simulink model "VAS_LEVEL1_TASK0_SETUP"  (Simulink 3.00)
undefined symbols (not defined in the file): data, dht, DHT_Z1, DHT_Z2, DHT_Z3, DHT_Z4, DHT_Z5, DHT_Z6, DHT_Z7, DHT_Z8, ephem, ephem_updater_bct, ephem_updater_ect, ephem_updater_moonrise, ephem_updater_moonset, ephem_updater_moontransit, ephem_updater_sunrise, ephem_updater_sunset, ephem_updater_suntransit, python, rex
libraries: mathlib x85, paramlib x18, logiclib x18, speclib x16, genlib x4, matrixlib x2, timelib x1

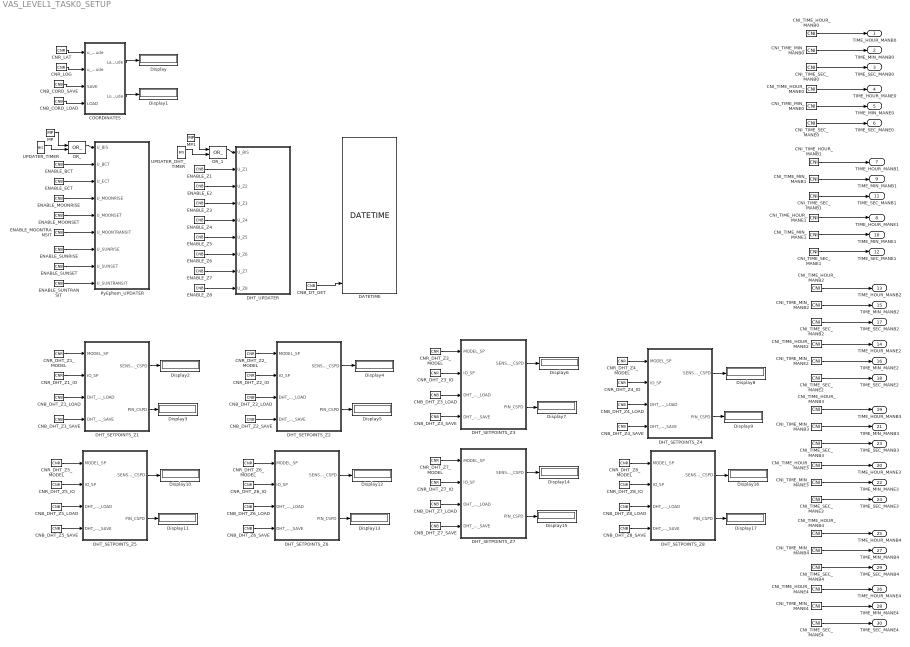
== system VAS_LEVEL1_TASK0_SETUP ==
  CNB_CORD_LOAD : mathlib/CNB  YCN=off
  CNB_CORD_SAVE : mathlib/CNB  YCN=off
  CNB_DHT_Z1_LOAD : mathlib/CNB  YCN=off
  CNB_DHT_Z1_SAVE : mathlib/CNB  YCN=off
  CNB_DHT_Z2_LOAD : mathlib/CNB  YCN=off
  CNB_DHT_Z2_SAVE : mathlib/CNB  YCN=off
  CNB_DHT_Z3_LOAD : mathlib/CNB  YCN=off
  CNB_DHT_Z3_SAVE : mathlib/CNB  YCN=off
  CNB_DHT_Z4_LOAD : mathlib/CNB  YCN=off
  CNB_DHT_Z4_SAVE : mathlib/CNB  YCN=off
  CNB_DHT_Z5_LOAD : mathlib/CNB  YCN=off
  CNB_DHT_Z5_SAVE : mathlib/CNB  YCN=off
  CNB_DHT_Z6_LOAD : mathlib/CNB  YCN=off
  CNB_DHT_Z6_SAVE : mathlib/CNB  YCN=off
  CNB_DHT_Z7_LOAD : mathlib/CNB  YCN=off
  CNB_DHT_Z7_SAVE : mathlib/CNB  YCN=off
  CNB_DHT_Z8_LOAD : mathlib/CNB  YCN=off
  CNB_DHT_Z8_SAVE : mathlib/CNB  YCN=off
  CNB_DT_GET : mathlib/CNB  YCN=off
  CNI_TIME_HOUR_MANB0 : mathlib/CNI  icn=20
  CNI_TIME_HOUR_MANB1 : mathlib/CNI  icn=14
  CNI_TIME_HOUR_MANB2 : mathlib/CNI  icn=16
  CNI_TIME_HOUR_MANB3 : mathlib/CNI  icn=18
  CNI_TIME_HOUR_MANB4 : mathlib/CNI  icn=0
  CNI_TIME_HOUR_MANE0 : mathlib/CNI  icn=22
  CNI_TIME_HOUR_MANE1 : mathlib/CNI  icn=16
  CNI_TIME_HOUR_MANE2 : mathlib/CNI  icn=18
  CNI_TIME_HOUR_MANE3 : mathlib/CNI  icn=20
  CNI_TIME_HOUR_MANE4 : mathlib/CNI  icn=0
  CNI_TIME_MIN_MANB{0..4} (5 alike) : mathlib/CNI  icn=0
  CNI_TIME_MIN_MANE{0..3} (4 alike) : mathlib/CNI  icn=0
  CNI_TIME_MIN_MANE4 : mathlib/CNI  icn=50
  CNI_TIME_SEC_MANB{0..4} (5 alike) : mathlib/CNI  icn=0
  CNI_TIME_SEC_MANE{0..4} (5 alike) : mathlib/CNI  icn=0
  CNR_DHT_Z1_IO : mathlib/CNR  ycn=5
  CNR_DHT_Z1_MODEL : mathlib/CNR  ycn=2
  CNR_DHT_Z2_IO : mathlib/CNR  ycn=6
  CNR_DHT_Z2_MODEL : mathlib/CNR  ycn=2
  CNR_DHT_Z3_IO : mathlib/CNR  ycn=16
  CNR_DHT_Z3_MODEL : mathlib/CNR  ycn=2
  CNR_DHT_Z4_IO : mathlib/CNR  ycn=17
  CNR_DHT_Z4_MODEL : mathlib/CNR  ycn=2
  CNR_DHT_Z5_IO : mathlib/CNR  ycn=0
  CNR_DHT_Z5_MODEL : mathlib/CNR  ycn=2
  CNR_DHT_Z6_IO : mathlib/CNR  ycn=0
  CNR_DHT_Z6_MODEL : mathlib/CNR  ycn=2
  CNR_DHT_Z7_IO : mathlib/CNR  ycn=0
  CNR_DHT_Z7_MODEL : mathlib/CNR  ycn=2
  CNR_DHT_Z8_IO : mathlib/CNR  ycn=0
  CNR_DHT_Z8_MODEL : mathlib/CNR  ycn=2
  CNR_LAT : mathlib/CNR  ycn=31.1729
  CNR_LOG : mathlib/CNR  ycn=-81.4772
  COORDINATES : Subsystem
      mask Type: REX sequence
  DATETIME : timelib/DATETIME  isetmode=6: The usec input - set HW clock only  igetmode=7: HW clock  settol=1  setper=0  getper=0.001  FDOW=off  tz=1: Local time
  DHT_SETPOINTS_Z1 : Subsystem
      mask Type: REX sequence
  DHT_SETPOINTS_Z2 : Subsystem
      mask Type: REX sequence
  DHT_SETPOINTS_Z3 : Subsystem
      mask Type: REX sequence
  DHT_SETPOINTS_Z4 : Subsystem
      mask Type: REX sequence
  DHT_SETPOINTS_Z5 : Subsystem
      mask Type: REX sequence
  DHT_SETPOINTS_Z6 : Subsystem
      mask Type: REX sequence
  DHT_SETPOINTS_Z7 : Subsystem
      mask Type: REX sequence
  DHT_SETPOINTS_Z8 : Subsystem
      mask Type: REX sequence
  DHT_UPDATER : Subsystem
      mask Type: REX sequence
  Display{,1..17} (18 alike) : Display
      settings: Format=Best fit
  ENABLE_BCT : mathlib/CNB  YCN=on
  ENABLE_E2 : mathlib/CNB  YCN=off
  ENABLE_ECT : mathlib/CNB  YCN=on
  ENABLE_MOONRISE : mathlib/CNB  YCN=on
  ENABLE_MOONSET : mathlib/CNB  YCN=on
  ENABLE_MOONTRANSIT : mathlib/CNB  YCN=on
  ENABLE_SUNRISE : mathlib/CNB  YCN=on
  ENABLE_SUNSET : mathlib/CNB  YCN=on
  ENABLE_SUNTRANSIT : mathlib/CNB  YCN=on
  ENABLE_Z{1,3..8} (7 alike) : mathlib/CNB  YCN=off
  MP : genlib/MP  BSTATE=on  pwidth=2  RPTF=off
  MP1 : genlib/MP  BSTATE=on  pwidth=2  RPTF=off
  OR_ : logiclib/OR_
  OR_1 : logiclib/OR_
  PyEphem_UPDATER : Subsystem
      mask Type: REX sequence
  UPDATER_DHT_TIMER : genlib/BIS  Y0=off  t1=0  t2=1  t3=15  t4=4  t5=5  t6=6  t7=7  t8=8  RPT=on  bEdit=off
  UPDATER_TIMER : genlib/BIS  Y0=off  t1=0  t2=1  t3=3600  t4=4  t5=5  t6=6  t7=7  t8=8  RPT=on  bEdit=off
  TIME_HOUR_MANB0 : Outport  Port=1
  TIME_MIN_MANB0 : Outport  Port=2
  TIME_SEC_MANB0 : Outport  Port=3
  TIME_HOUR_MANE0 : Outport  Port=4
  TIME_MIN_MANE0 : Outport  Port=5
  TIME_SEC_MANE0 : Outport  Port=6
  TIME_HOUR_MANB1 : Outport  Port=7
  TIME_HOUR_MANE1 : Outport  Port=8
  TIME_MIN_MANB1 : Outport  Port=9
  TIME_MIN_MANE1 : Outport  Port=10
  TIME_SEC_MANB1 : Outport  Port=11
  TIME_SEC_MANE1 : Outport  Port=12
  TIME_HOUR_MANB2 : Outport  Port=13
  TIME_HOUR_MANE2 : Outport  Port=14
  TIME_MIN_MANB2 : Outport  Port=15
  TIME_MIN_MANE2 : Outport  Port=16
  TIME_SEC_MANB2 : Outport  Port=17
  TIME_SEC_MANE2 : Outport  Port=18
  TIME_HOUR_MANB3 : Outport  Port=19
  TIME_HOUR_MANE3 : Outport  Port=20
  TIME_MIN_MANB3 : Outport  Port=21
  TIME_MIN_MANE3 : Outport  Port=22
  TIME_SEC_MANB3 : Outport  Port=23
  TIME_SEC_MANE3 : Outport  Port=24
  TIME_HOUR_MANB4 : Outport  Port=25
  TIME_HOUR_MANE4 : Outport  Port=26
  TIME_MIN_MANB4 : Outport  Port=27
  TIME_MIN_MANE4 : Outport  Port=28
  TIME_SEC_MANB4 : Outport  Port=29
  TIME_SEC_MANE4 : Outport  Port=30
  wires:
  CNB_CORD_LOAD/1 -> COORDINATES/4(LOAD)
  CNB_CORD_SAVE/1 -> COORDINATES/3(SAVE)
  CNB_DHT_Z1_LOAD/1 -> DHT_SETPOINTS_Z1/3(DHT_MIO_LOAD)
  CNB_DHT_Z1_SAVE/1 -> DHT_SETPOINTS_Z1/4(DHT_MIO_SAVE)
  CNB_DHT_Z2_LOAD/1 -> DHT_SETPOINTS_Z2/3(DHT_MIO_LOAD)
  CNB_DHT_Z2_SAVE/1 -> DHT_SETPOINTS_Z2/4(DHT_MIO_SAVE)
  CNB_DHT_Z3_LOAD/1 -> DHT_SETPOINTS_Z3/3(DHT_MIO_LOAD)
  CNB_DHT_Z3_SAVE/1 -> DHT_SETPOINTS_Z3/4(DHT_MIO_SAVE)
  CNB_DHT_Z4_LOAD/1 -> DHT_SETPOINTS_Z4/3(DHT_MIO_LOAD)
  CNB_DHT_Z4_SAVE/1 -> DHT_SETPOINTS_Z4/4(DHT_MIO_SAVE)
  CNB_DHT_Z5_LOAD/1 -> DHT_SETPOINTS_Z5/3(DHT_MIO_LOAD)
  CNB_DHT_Z5_SAVE/1 -> DHT_SETPOINTS_Z5/4(DHT_MIO_SAVE)
  CNB_DHT_Z6_LOAD/1 -> DHT_SETPOINTS_Z6/3(DHT_MIO_LOAD)
  CNB_DHT_Z6_SAVE/1 -> DHT_SETPOINTS_Z6/4(DHT_MIO_SAVE)
  CNB_DHT_Z7_LOAD/1 -> DHT_SETPOINTS_Z7/3(DHT_MIO_LOAD)
  CNB_DHT_Z7_SAVE/1 -> DHT_SETPOINTS_Z7/4(DHT_MIO_SAVE)
  CNB_DHT_Z8_LOAD/1 -> DHT_SETPOINTS_Z8/3(DHT_MIO_LOAD)
  CNB_DHT_Z8_SAVE/1 -> DHT_SETPOINTS_Z8/4(DHT_MIO_SAVE)
  CNB_DT_GET/1 -> DATETIME/9
  CNI_TIME_HOUR_MANB0/1 -> TIME_HOUR_MANB0/1
  CNI_TIME_HOUR_MANB1/1 -> TIME_HOUR_MANB1/1
  CNI_TIME_HOUR_MANB2/1 -> TIME_HOUR_MANB2/1
  CNI_TIME_HOUR_MANB3/1 -> TIME_HOUR_MANB3/1
  CNI_TIME_HOUR_MANB4/1 -> TIME_HOUR_MANB4/1
  CNI_TIME_HOUR_MANE0/1 -> TIME_HOUR_MANE0/1
  CNI_TIME_HOUR_MANE1/1 -> TIME_HOUR_MANE1/1
  CNI_TIME_HOUR_MANE2/1 -> TIME_HOUR_MANE2/1
  CNI_TIME_HOUR_MANE3/1 -> TIME_HOUR_MANE3/1
  CNI_TIME_HOUR_MANE4/1 -> TIME_HOUR_MANE4/1
  CNI_TIME_MIN_MANB0/1 -> TIME_MIN_MANB0/1
  CNI_TIME_MIN_MANB1/1 -> TIME_MIN_MANB1/1
  CNI_TIME_MIN_MANB2/1 -> TIME_MIN_MANB2/1
  CNI_TIME_MIN_MANB3/1 -> TIME_MIN_MANB3/1
  CNI_TIME_MIN_MANB4/1 -> TIME_MIN_MANB4/1
  CNI_TIME_MIN_MANE0/1 -> TIME_MIN_MANE0/1
  CNI_TIME_MIN_MANE1/1 -> TIME_MIN_MANE1/1
  CNI_TIME_MIN_MANE2/1 -> TIME_MIN_MANE2/1
  CNI_TIME_MIN_MANE3/1 -> TIME_MIN_MANE3/1
  CNI_TIME_MIN_MANE4/1 -> TIME_MIN_MANE4/1
  CNI_TIME_SEC_MANB0/1 -> TIME_SEC_MANB0/1
  CNI_TIME_SEC_MANB1/1 -> TIME_SEC_MANB1/1
  CNI_TIME_SEC_MANB2/1 -> TIME_SEC_MANB2/1
  CNI_TIME_SEC_MANB3/1 -> TIME_SEC_MANB3/1
  CNI_TIME_SEC_MANB4/1 -> TIME_SEC_MANB4/1
  CNI_TIME_SEC_MANE0/1 -> TIME_SEC_MANE0/1
  CNI_TIME_SEC_MANE1/1 -> TIME_SEC_MANE1/1
  CNI_TIME_SEC_MANE2/1 -> TIME_SEC_MANE2/1
  CNI_TIME_SEC_MANE3/1 -> TIME_SEC_MANE3/1
  CNI_TIME_SEC_MANE4/1 -> TIME_SEC_MANE4/1
  CNR_DHT_Z1_IO/1 -> DHT_SETPOINTS_Z1/2(IO_SP)
  CNR_DHT_Z1_MODEL/1 -> DHT_SETPOINTS_Z1/1(MODEL_SP)
  CNR_DHT_Z2_IO/1 -> DHT_SETPOINTS_Z2/2(IO_SP)
  CNR_DHT_Z2_MODEL/1 -> DHT_SETPOINTS_Z2/1(MODEL_SP)
  CNR_DHT_Z3_IO/1 -> DHT_SETPOINTS_Z3/2(IO_SP)
  CNR_DHT_Z3_MODEL/1 -> DHT_SETPOINTS_Z3/1(MODEL_SP)
  CNR_DHT_Z4_IO/1 -> DHT_SETPOINTS_Z4/2(IO_SP)
  CNR_DHT_Z4_MODEL/1 -> DHT_SETPOINTS_Z4/1(MODEL_SP)
  CNR_DHT_Z5_IO/1 -> DHT_SETPOINTS_Z5/2(IO_SP)
  CNR_DHT_Z5_MODEL/1 -> DHT_SETPOINTS_Z5/1(MODEL_SP)
  CNR_DHT_Z6_IO/1 -> DHT_SETPOINTS_Z6/2(IO_SP)
  CNR_DHT_Z6_MODEL/1 -> DHT_SETPOINTS_Z6/1(MODEL_SP)
  CNR_DHT_Z7_IO/1 -> DHT_SETPOINTS_Z7/2(IO_SP)
  CNR_DHT_Z7_MODEL/1 -> DHT_SETPOINTS_Z7/1(MODEL_SP)
  CNR_DHT_Z8_IO/1 -> DHT_SETPOINTS_Z8/2(IO_SP)
  CNR_DHT_Z8_MODEL/1 -> DHT_SETPOINTS_Z8/1(MODEL_SP)
  CNR_LAT/1 -> COORDINATES/1(u_Latitude)
  CNR_LOG/1 -> COORDINATES/2(u_Longitude)
  COORDINATES/1(Latitude) -> Display/1
  COORDINATES/2(Longitude) -> Display1/1
  DHT_SETPOINTS_Z1/1(SENSOR_CSPD) -> Display2/1
  DHT_SETPOINTS_Z1/2(PIN_CSPD) -> Display3/1
  DHT_SETPOINTS_Z2/1(SENSOR_CSPD) -> Display4/1
  DHT_SETPOINTS_Z2/2(PIN_CSPD) -> Display5/1
  DHT_SETPOINTS_Z3/1(SENSOR_CSPD) -> Display6/1
  DHT_SETPOINTS_Z3/2(PIN_CSPD) -> Display7/1
  DHT_SETPOINTS_Z4/1(SENSOR_CSPD) -> Display8/1
  DHT_SETPOINTS_Z4/2(PIN_CSPD) -> Display9/1
  DHT_SETPOINTS_Z5/1(SENSOR_CSPD) -> Display10/1
  DHT_SETPOINTS_Z5/2(PIN_CSPD) -> Display11/1
  DHT_SETPOINTS_Z6/1(SENSOR_CSPD) -> Display12/1
  DHT_SETPOINTS_Z6/2(PIN_CSPD) -> Display13/1
  DHT_SETPOINTS_Z7/1(SENSOR_CSPD) -> Display14/1
  DHT_SETPOINTS_Z7/2(PIN_CSPD) -> Display15/1
  DHT_SETPOINTS_Z8/1(SENSOR_CSPD) -> Display16/1
  DHT_SETPOINTS_Z8/2(PIN_CSPD) -> Display17/1
  ENABLE_BCT/1 -> PyEphem_UPDATER/2(U_BCT)
  ENABLE_E2/1 -> DHT_UPDATER/3(U_Z2)
  ENABLE_ECT/1 -> PyEphem_UPDATER/3(U_ECT)
  ENABLE_MOONRISE/1 -> PyEphem_UPDATER/4(U_MOONRISE)
  ENABLE_MOONSET/1 -> PyEphem_UPDATER/5(U_MOONSET)
  ENABLE_MOONTRANSIT/1 -> PyEphem_UPDATER/6(U_MOONTRANSIT)
  ENABLE_SUNRISE/1 -> PyEphem_UPDATER/7(U_SUNRISE)
  ENABLE_SUNSET/1 -> PyEphem_UPDATER/8(U_SUNSET)
  ENABLE_SUNTRANSIT/1 -> PyEphem_UPDATER/9(U_SUNTRANSIT)
  ENABLE_Z1/1 -> DHT_UPDATER/2(U_Z1)
  ENABLE_Z3/1 -> DHT_UPDATER/4(U_Z3)
  ENABLE_Z4/1 -> DHT_UPDATER/5(U_Z4)
  ENABLE_Z5/1 -> DHT_UPDATER/6(U_Z5)
  ENABLE_Z6/1 -> DHT_UPDATER/7(U_Z6)
  ENABLE_Z7/1 -> DHT_UPDATER/8(U_Z7)
  ENABLE_Z8/1 -> DHT_UPDATER/9(U_Z8)
  MP/1 -> OR_/1
  MP1/1 -> OR_1/1
  OR_/1 -> PyEphem_UPDATER/1(U_BIS)
  OR_1/1 -> DHT_UPDATER/1(U_BIS)
  UPDATER_DHT_TIMER/1 -> OR_1/2
  UPDATER_TIMER/1 -> OR_/2

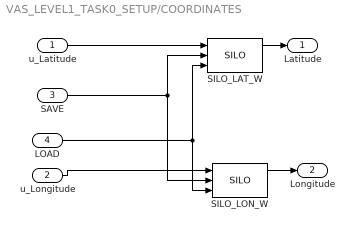
== system VAS_LEVEL1_TASK0_SETUP/COORDINATES ==
  u_Latitude : Inport  Port=1
  u_Longitude : Inport  Port=2
  SAVE : Inport  Port=3
  LOAD : Inport  Port=4
  SILO_LAT_W : paramlib/SILO  fname=/static/LAT.txt  CSF=off  CLF=off  yerr=0
  SILO_LON_W : paramlib/SILO  fname=/static/LON.txt  CSF=off  CLF=off  yerr=0
  Latitude : Outport  Port=1
  Longitude : Outport  Port=2
  wires:
  LOAD/1 -> SILO_LAT_W/3, SILO_LON_W/3
  SAVE/1 -> SILO_LAT_W/2, SILO_LON_W/2
  SILO_LAT_W/1 -> Latitude/1
  SILO_LON_W/1 -> Longitude/1
  u_Latitude/1 -> SILO_LAT_W/1
  u_Longitude/1 -> SILO_LON_W/1

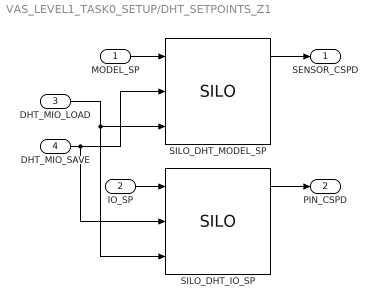
== system VAS_LEVEL1_TASK0_SETUP/DHT_SETPOINTS_Z1 ==
  MODEL_SP : Inport  Port=1
  IO_SP : Inport  Port=2
  DHT_MIO_LOAD : Inport  Port=3
  DHT_MIO_SAVE : Inport  Port=4
  SILO_DHT_IO_SP : paramlib/SILO  fname=/static/DHT_Z1_PIN.txt  CSF=off  CLF=off  yerr=0
  SILO_DHT_MODEL_SP : paramlib/SILO  fname=/static/DHT_Z1_SENSOR.txt  CSF=off  CLF=off  yerr=0
  SENSOR_CSPD : Outport  Port=1
  PIN_CSPD : Outport  Port=2
  wires:
  DHT_MIO_LOAD/1 -> SILO_DHT_IO_SP/3, SILO_DHT_MODEL_SP/3
  DHT_MIO_SAVE/1 -> SILO_DHT_IO_SP/2, SILO_DHT_MODEL_SP/2
  IO_SP/1 -> SILO_DHT_IO_SP/1
  MODEL_SP/1 -> SILO_DHT_MODEL_SP/1
  SILO_DHT_IO_SP/1 -> PIN_CSPD/1
  SILO_DHT_MODEL_SP/1 -> SENSOR_CSPD/1

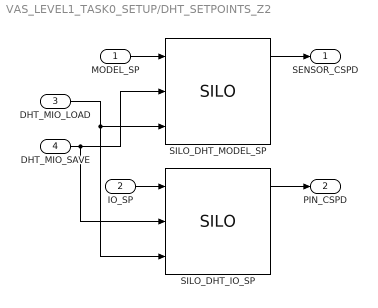
== system VAS_LEVEL1_TASK0_SETUP/DHT_SETPOINTS_Z2 ==
  MODEL_SP : Inport  Port=1
  IO_SP : Inport  Port=2
  DHT_MIO_LOAD : Inport  Port=3
  DHT_MIO_SAVE : Inport  Port=4
  SILO_DHT_IO_SP : paramlib/SILO  fname=/static/DHT_Z2_PIN.txt  CSF=off  CLF=off  yerr=0
  SILO_DHT_MODEL_SP : paramlib/SILO  fname=/static/DHT_Z2_SENSOR.txt  CSF=off  CLF=off  yerr=0
  SENSOR_CSPD : Outport  Port=1
  PIN_CSPD : Outport  Port=2
  wires:
  DHT_MIO_LOAD/1 -> SILO_DHT_IO_SP/3, SILO_DHT_MODEL_SP/3
  DHT_MIO_SAVE/1 -> SILO_DHT_IO_SP/2, SILO_DHT_MODEL_SP/2
  IO_SP/1 -> SILO_DHT_IO_SP/1
  MODEL_SP/1 -> SILO_DHT_MODEL_SP/1
  SILO_DHT_IO_SP/1 -> PIN_CSPD/1
  SILO_DHT_MODEL_SP/1 -> SENSOR_CSPD/1

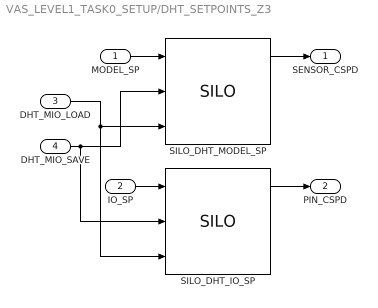
== system VAS_LEVEL1_TASK0_SETUP/DHT_SETPOINTS_Z3 ==
  MODEL_SP : Inport  Port=1
  IO_SP : Inport  Port=2
  DHT_MIO_LOAD : Inport  Port=3
  DHT_MIO_SAVE : Inport  Port=4
  SILO_DHT_IO_SP : paramlib/SILO  fname=/static/DHT_Z3_PIN.txt  CSF=off  CLF=off  yerr=0
  SILO_DHT_MODEL_SP : paramlib/SILO  fname=/static/DHT_Z3_SENSOR.txt  CSF=off  CLF=off  yerr=0
  SENSOR_CSPD : Outport  Port=1
  PIN_CSPD : Outport  Port=2
  wires:
  DHT_MIO_LOAD/1 -> SILO_DHT_IO_SP/3, SILO_DHT_MODEL_SP/3
  DHT_MIO_SAVE/1 -> SILO_DHT_IO_SP/2, SILO_DHT_MODEL_SP/2
  IO_SP/1 -> SILO_DHT_IO_SP/1
  MODEL_SP/1 -> SILO_DHT_MODEL_SP/1
  SILO_DHT_IO_SP/1 -> PIN_CSPD/1
  SILO_DHT_MODEL_SP/1 -> SENSOR_CSPD/1

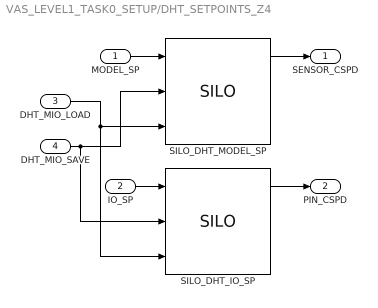
== system VAS_LEVEL1_TASK0_SETUP/DHT_SETPOINTS_Z4 ==
  MODEL_SP : Inport  Port=1
  IO_SP : Inport  Port=2
  DHT_MIO_LOAD : Inport  Port=3
  DHT_MIO_SAVE : Inport  Port=4
  SILO_DHT_IO_SP : paramlib/SILO  fname=/static/DHT_Z4_PIN.txt  CSF=off  CLF=off  yerr=0
  SILO_DHT_MODEL_SP : paramlib/SILO  fname=/static/DHT_Z4_SENSOR.txt  CSF=off  CLF=off  yerr=0
  SENSOR_CSPD : Outport  Port=1
  PIN_CSPD : Outport  Port=2
  wires:
  DHT_MIO_LOAD/1 -> SILO_DHT_IO_SP/3, SILO_DHT_MODEL_SP/3
  DHT_MIO_SAVE/1 -> SILO_DHT_IO_SP/2, SILO_DHT_MODEL_SP/2
  IO_SP/1 -> SILO_DHT_IO_SP/1
  MODEL_SP/1 -> SILO_DHT_MODEL_SP/1
  SILO_DHT_IO_SP/1 -> PIN_CSPD/1
  SILO_DHT_MODEL_SP/1 -> SENSOR_CSPD/1

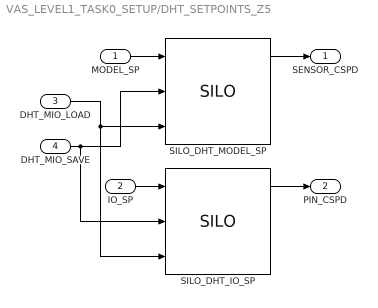
== system VAS_LEVEL1_TASK0_SETUP/DHT_SETPOINTS_Z5 ==
  MODEL_SP : Inport  Port=1
  IO_SP : Inport  Port=2
  DHT_MIO_LOAD : Inport  Port=3
  DHT_MIO_SAVE : Inport  Port=4
  SILO_DHT_IO_SP : paramlib/SILO  fname=/static/DHT_Z5_PIN.txt  CSF=off  CLF=off  yerr=0
  SILO_DHT_MODEL_SP : paramlib/SILO  fname=/static/DHT_Z5_SENSOR.txt  CSF=off  CLF=off  yerr=0
  SENSOR_CSPD : Outport  Port=1
  PIN_CSPD : Outport  Port=2
  wires:
  DHT_MIO_LOAD/1 -> SILO_DHT_IO_SP/3, SILO_DHT_MODEL_SP/3
  DHT_MIO_SAVE/1 -> SILO_DHT_IO_SP/2, SILO_DHT_MODEL_SP/2
  IO_SP/1 -> SILO_DHT_IO_SP/1
  MODEL_SP/1 -> SILO_DHT_MODEL_SP/1
  SILO_DHT_IO_SP/1 -> PIN_CSPD/1
  SILO_DHT_MODEL_SP/1 -> SENSOR_CSPD/1

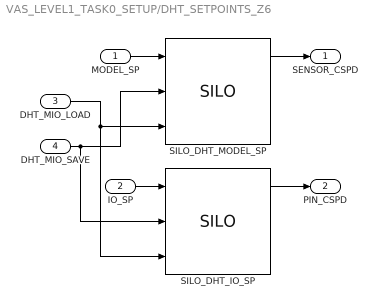
== system VAS_LEVEL1_TASK0_SETUP/DHT_SETPOINTS_Z6 ==
  MODEL_SP : Inport  Port=1
  IO_SP : Inport  Port=2
  DHT_MIO_LOAD : Inport  Port=3
  DHT_MIO_SAVE : Inport  Port=4
  SILO_DHT_IO_SP : paramlib/SILO  fname=/static/DHT_Z6_PIN.txt  CSF=off  CLF=off  yerr=0
  SILO_DHT_MODEL_SP : paramlib/SILO  fname=/static/DHT_Z6_SENSOR.txt  CSF=off  CLF=off  yerr=0
  SENSOR_CSPD : Outport  Port=1
  PIN_CSPD : Outport  Port=2
  wires:
  DHT_MIO_LOAD/1 -> SILO_DHT_IO_SP/3, SILO_DHT_MODEL_SP/3
  DHT_MIO_SAVE/1 -> SILO_DHT_IO_SP/2, SILO_DHT_MODEL_SP/2
  IO_SP/1 -> SILO_DHT_IO_SP/1
  MODEL_SP/1 -> SILO_DHT_MODEL_SP/1
  SILO_DHT_IO_SP/1 -> PIN_CSPD/1
  SILO_DHT_MODEL_SP/1 -> SENSOR_CSPD/1

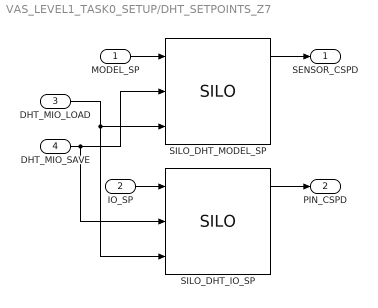
== system VAS_LEVEL1_TASK0_SETUP/DHT_SETPOINTS_Z7 ==
  MODEL_SP : Inport  Port=1
  IO_SP : Inport  Port=2
  DHT_MIO_LOAD : Inport  Port=3
  DHT_MIO_SAVE : Inport  Port=4
  SILO_DHT_IO_SP : paramlib/SILO  fname=/static/DHT_Z7_PIN.txt  CSF=off  CLF=off  yerr=0
  SILO_DHT_MODEL_SP : paramlib/SILO  fname=/static/DHT_Z7_SENSOR.txt  CSF=off  CLF=off  yerr=0
  SENSOR_CSPD : Outport  Port=1
  PIN_CSPD : Outport  Port=2
  wires:
  DHT_MIO_LOAD/1 -> SILO_DHT_IO_SP/3, SILO_DHT_MODEL_SP/3
  DHT_MIO_SAVE/1 -> SILO_DHT_IO_SP/2, SILO_DHT_MODEL_SP/2
  IO_SP/1 -> SILO_DHT_IO_SP/1
  MODEL_SP/1 -> SILO_DHT_MODEL_SP/1
  SILO_DHT_IO_SP/1 -> PIN_CSPD/1
  SILO_DHT_MODEL_SP/1 -> SENSOR_CSPD/1

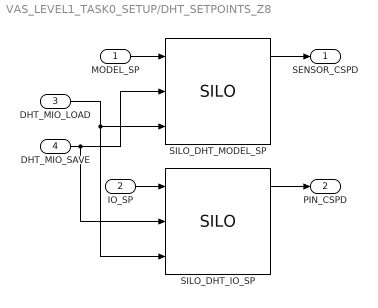
== system VAS_LEVEL1_TASK0_SETUP/DHT_SETPOINTS_Z8 ==
  MODEL_SP : Inport  Port=1
  IO_SP : Inport  Port=2
  DHT_MIO_LOAD : Inport  Port=3
  DHT_MIO_SAVE : Inport  Port=4
  SILO_DHT_IO_SP : paramlib/SILO  fname=/static/DHT_Z8_PIN.txt  CSF=off  CLF=off  yerr=0
  SILO_DHT_MODEL_SP : paramlib/SILO  fname=/static/DHT_Z8_SENSOR.txt  CSF=off  CLF=off  yerr=0
  SENSOR_CSPD : Outport  Port=1
  PIN_CSPD : Outport  Port=2
  wires:
  DHT_MIO_LOAD/1 -> SILO_DHT_IO_SP/3, SILO_DHT_MODEL_SP/3
  DHT_MIO_SAVE/1 -> SILO_DHT_IO_SP/2, SILO_DHT_MODEL_SP/2
  IO_SP/1 -> SILO_DHT_IO_SP/1
  MODEL_SP/1 -> SILO_DHT_MODEL_SP/1
  SILO_DHT_IO_SP/1 -> PIN_CSPD/1
  SILO_DHT_MODEL_SP/1 -> SENSOR_CSPD/1

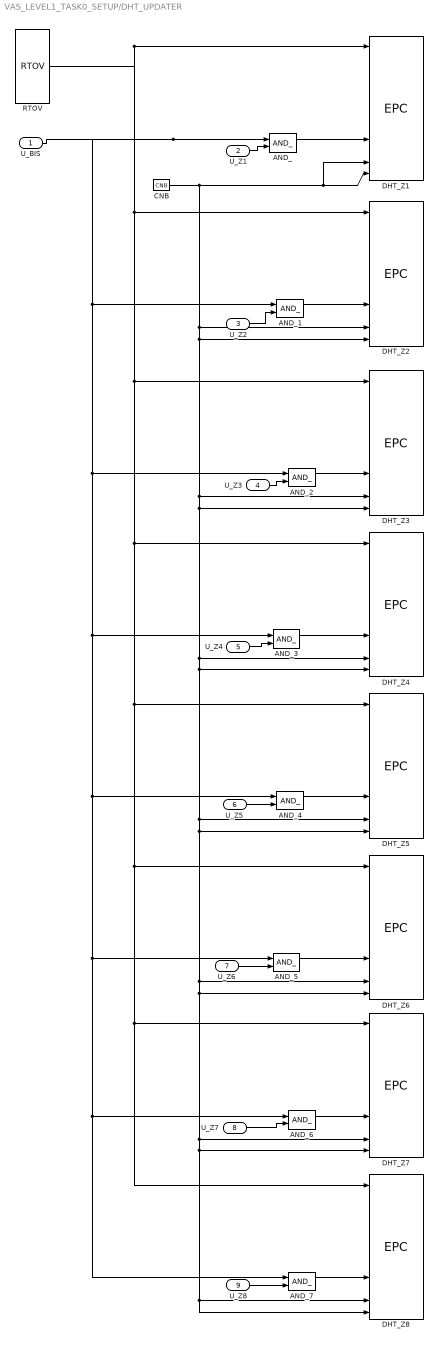
== system VAS_LEVEL1_TASK0_SETUP/DHT_UPDATER ==
  U_BIS : Inport  Port=1
  U_Z1 : Inport  Port=2
  U_Z2 : Inport  Port=3
  U_Z3 : Inport  Port=4
  U_Z4 : Inport  Port=5
  U_Z5 : Inport  Port=6
  U_Z6 : Inport  Port=7
  U_Z7 : Inport  Port=8
  U_Z8 : Inport  Port=9
  AND_{,1..7} (8 alike) : logiclib/AND_
  CNB : mathlib/CNB  YCN=off
  DHT_Z1 : speclib/EPC  cmd=python /rex/data/dht/DHT_Z1.py  sl=0  ifm=1  format=1: Space-delimited values  nmax=2
  DHT_Z2 : speclib/EPC  cmd=python /rex/data/dht/DHT_Z2.py  sl=0  ifm=1  format=1: Space-delimited values  nmax=2
  DHT_Z3 : speclib/EPC  cmd=python /rex/data/dht/DHT_Z3.py  sl=0  ifm=1  format=1: Space-delimited values  nmax=2
  DHT_Z4 : speclib/EPC  cmd=python /rex/data/dht/DHT_Z4.py  sl=0  ifm=1  format=1: Space-delimited values  nmax=2
  DHT_Z5 : speclib/EPC  cmd=python /rex/data/dht/DHT_Z5.py  sl=0  ifm=1  format=1: Space-delimited values  nmax=2
  DHT_Z6 : speclib/EPC  cmd=python /rex/data/dht/DHT_Z6.py  sl=0  ifm=1  format=1: Space-delimited values  nmax=2
  DHT_Z7 : speclib/EPC  cmd=python /rex/data/dht/DHT_Z7.py  sl=0  ifm=1  format=1: Space-delimited values  nmax=2
  DHT_Z8 : speclib/EPC  cmd=python /rex/data/dht/DHT_Z8.py  sl=0  ifm=1  format=1: Space-delimited values  nmax=2
  RTOV : matrixlib/RTOV  nmax=8  offset=0  n=8  etype=8: Double
  wires:
  AND_/1 -> DHT_Z1/9
  AND_1/1 -> DHT_Z2/9
  AND_2/1 -> DHT_Z3/9
  AND_3/1 -> DHT_Z4/9
  AND_4/1 -> DHT_Z5/9
  AND_5/1 -> DHT_Z6/9
  AND_6/1 -> DHT_Z7/9
  AND_7/1 -> DHT_Z8/9
  CNB/1 -> DHT_Z1/11, DHT_Z1/12, DHT_Z2/11, DHT_Z2/12, DHT_Z3/11, DHT_Z3/12, DHT_Z4/11, DHT_Z4/12, DHT_Z5/11, DHT_Z5/12, DHT_Z6/11, DHT_Z6/12, DHT_Z7/11, DHT_Z7/12, DHT_Z8/11, DHT_Z8/12
  RTOV/1 -> DHT_Z1/1, DHT_Z2/1, DHT_Z7/1, DHT_Z8/1, DHT_Z6/1, DHT_Z5/1, DHT_Z4/1, DHT_Z3/1
  U_BIS/1 -> AND_/1, AND_1/1, AND_5/1, AND_6/1, AND_7/1, AND_4/1, AND_3/1, AND_2/1
  U_Z1/1 -> AND_/2
  U_Z2/1 -> AND_1/2
  U_Z3/1 -> AND_2/2
  U_Z4/1 -> AND_3/2
  U_Z5/1 -> AND_4/2
  U_Z6/1 -> AND_5/2
  U_Z7/1 -> AND_6/2
  U_Z8/1 -> AND_7/2

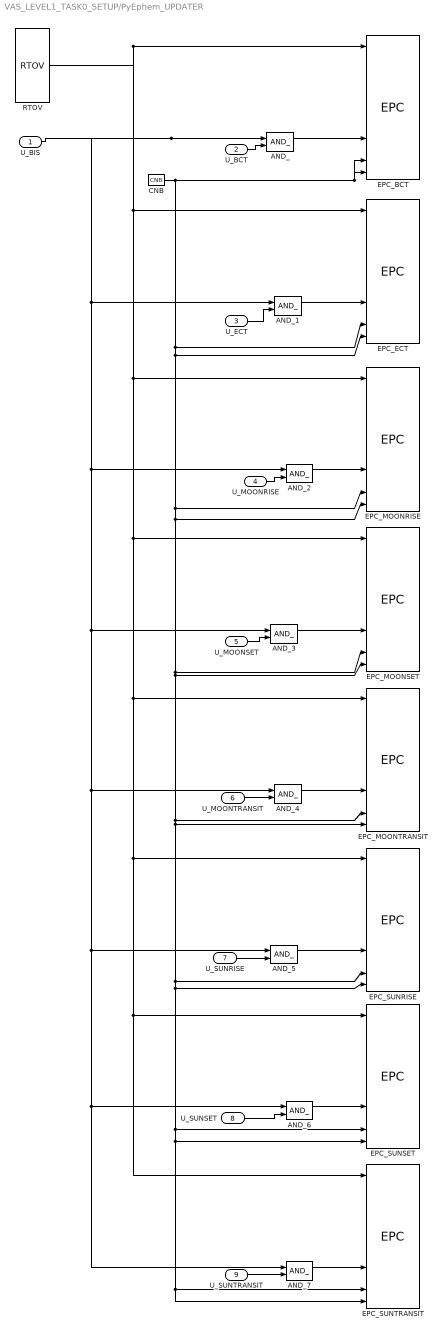
== system VAS_LEVEL1_TASK0_SETUP/PyEphem_UPDATER ==
  U_BIS : Inport  Port=1
  U_BCT : Inport  Port=2
  U_ECT : Inport  Port=3
  U_MOONRISE : Inport  Port=4
  U_MOONSET : Inport  Port=5
  U_MOONTRANSIT : Inport  Port=6
  U_SUNRISE : Inport  Port=7
  U_SUNSET : Inport  Port=8
  U_SUNTRANSIT : Inport  Port=9
  AND_{,1..7} (8 alike) : logiclib/AND_
  CNB : mathlib/CNB  YCN=off
  EPC_BCT : speclib/EPC  cmd=python /rex/data/ephem/ephem_updater_bct.py  sl=0  ifm=1  format=1: Space-delimited values  nmax=2
  EPC_ECT : speclib/EPC  cmd=python /rex/data/ephem/ephem_updater_ect.py  sl=0  ifm=1  format=1: Space-delimited values  nmax=2
  EPC_MOONRISE : speclib/EPC  cmd=python /rex/data/ephem/ephem_updater_moonrise.py  sl=0  ifm=1  format=1: Space-delimited values  nmax=2
  EPC_MOONSET : speclib/EPC  cmd=python /rex/data/ephem/ephem_updater_moonset.py  sl=0  ifm=1  format=1: Space-delimited values  nmax=2
  EPC_MOONTRANSIT : speclib/EPC  cmd=python /rex/data/ephem/ephem_updater_moontransit.py  sl=0  format=1: Space-delimited values  nmax=2
  EPC_SUNRISE : speclib/EPC  cmd=python /rex/data/ephem/ephem_updater_sunrise.py  sl=0  ifm=1  format=1: Space-delimited values  nmax=2
  EPC_SUNSET : speclib/EPC  cmd=python /rex/data/ephem/ephem_updater_sunset.py  sl=0  ifm=1  format=1: Space-delimited values  nmax=2
  EPC_SUNTRANSIT : speclib/EPC  cmd=python /rex/data/ephem/ephem_updater_suntransit.py  sl=0  ifm=1  format=1: Space-delimited values  nmax=2
  RTOV : matrixlib/RTOV  nmax=8  offset=0  n=8  etype=8: Double
  wires:
  AND_/1 -> EPC_BCT/9
  AND_1/1 -> EPC_ECT/9
  AND_2/1 -> EPC_MOONRISE/9
  AND_3/1 -> EPC_MOONSET/9
  AND_4/1 -> EPC_MOONTRANSIT/9
  AND_5/1 -> EPC_SUNRISE/9
  AND_6/1 -> EPC_SUNSET/9
  AND_7/1 -> EPC_SUNTRANSIT/9
  CNB/1 -> EPC_BCT/11, EPC_BCT/12, EPC_SUNTRANSIT/11, EPC_SUNTRANSIT/12, EPC_SUNSET/12, EPC_SUNSET/11, EPC_SUNRISE/12, EPC_SUNRISE/11, EPC_MOONTRANSIT/12, EPC_MOONTRANSIT/11, EPC_MOONSET/12, EPC_MOONSET/11, EPC_MOONRISE/12, EPC_MOONRISE/11, EPC_ECT/12, EPC_ECT/11
  RTOV/1 -> EPC_BCT/1, EPC_ECT/1, EPC_SUNSET/1, EPC_SUNTRANSIT/1, EPC_SUNRISE/1, EPC_MOONTRANSIT/1, EPC_MOONSET/1, EPC_MOONRISE/1
  U_BCT/1 -> AND_/2
  U_BIS/1 -> AND_/1, AND_1/1, AND_5/1, AND_6/1, AND_7/1, AND_4/1, AND_3/1, AND_2/1
  U_ECT/1 -> AND_1/2
  U_MOONRISE/1 -> AND_2/2
  U_MOONSET/1 -> AND_3/2
  U_MOONTRANSIT/1 -> AND_4/2
  U_SUNRISE/1 -> AND_5/2
  U_SUNSET/1 -> AND_6/2
  U_SUNTRANSIT/1 -> AND_7/2
